simulink model "PID_ros"  (R2017b)
settings: Solver=FixedStepAuto  StartTime=0.0  StopTime=inf  FixedStep=dt_ros  RelTol=1e-3
values from neighbouring files (symbols this model uses):
  dt_ros = 0.02    [DOB_ros_adaptive_setup.m]    (also in DOB_ros_adaptive_w_kappa_setup.m; DOB_ros_setup.m)
  dt_ros_single = single(0.02)    [DOB_ros_adaptive_setup.m]    (also in DOB_ros_adaptive_w_kappa_setup.m; DOB_ros_setup.m)
  kc11 = single(0.3)    [DOB_ros_adaptive_setup.m]    (also in DOB_ros_adaptive_w_kappa_setup.m = single(1); DOB_ros_setup.m = kc1)
  kc12 = single(1)    [DOB_ros_adaptive_setup.m]    (also in DOB_ros_adaptive_w_kappa_setup.m = single(0); DOB_ros_setup.m = 1)
  kc2 = single(0.25)    [DOB_ros_adaptive_setup.m]    (also in DOB_ros_adaptive_w_kappa_setup.m = single(0.5); DOB_ros_setup.m = single(0.1))
  steering_ratio = 14.8    [DOB_ros_adaptive_setup.m]    (also in DOB_ros_adaptive_w_kappa_setup.m; DOB_ros_setup.m)
undefined symbols (not defined in the file or in its folder): Enable, SteeringWheelAngleCmd, SteeringWheelAngleVelocity
libraries: robotlib x4
settings Model: Creator=chen_tang  LastModifiedBy=root
settings OptimizationCC: PassReuseOutputArgsThreshold=0  MaxStackSize=64
settings DebuggingCC: ParameterTunabilityLossMsg=error
settings HardwareCC: ProdBitPerPointer=32  ProdBitPerSizeT=32  ProdBitPerPtrDiffT=32  ProdLargestAtomicFloat=None  ProdIntDivRoundTo=Undefined  ProdEndianess=Unspecified  ProdWordSize=32  ProdHWDeviceType=Generic->Unspecified (assume 32-bit Generic)  UseEmbeddedCoderFeatures=off
settings SFSimCC: MATLABDynamicMemAlloc=off
settings RTWCC: SystemTargetFile=ert.tlc  HardwareBoard=Robot Operating System (ROS)  TemplateMakefile=ert_default_tmf  GenerateReport=on  Toolchain=Catkin  LaunchReport=on  TargetLang=C++
settings CodeAppCC: ForceParamTrailComments=on  OperatorAnnotations=on  StateflowObjectComments=on  MATLABSourceComments=on
settings ERTTargetCC: ERTCustomFileBanners=off  SupportContinuousTime=on  SupportNonInlinedSFcns=on  RemoveResetFunc=off  ModelStepFunctionPrototypeControlCompliant=off

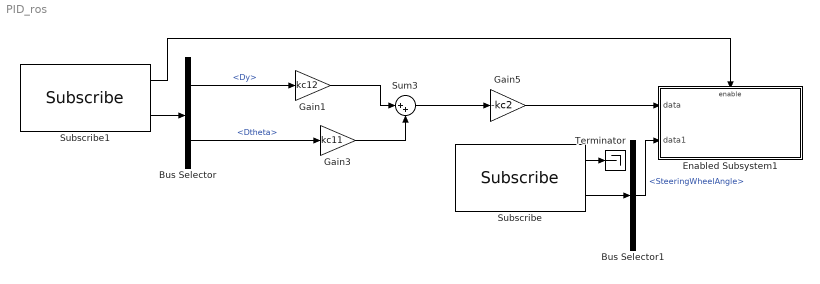
== system PID_ros ==
  Bus Selector : BusSelector  OutputSignals=Dy,Dtheta
  Bus Selector1 : BusSelector  OutputSignals=SteeringWheelAngle
  Enabled Subsystem1 : Subsystem  TreatAsAtomicUnit=on
  Gain1 : Gain  Gain=kc12  OutDataTypeStr=single
  Gain3 : Gain  Gain=kc11  OutDataTypeStr=single
  Gain5 : Gain  Gain=-kc2
  Subscribe : robotlib/Subscribe  SourceLibraryInfo=This block requires Robotics System Toolbox  topicSource=Specify your own  topic=/vehicle/steering_report  messageType=dbw_mkz_msgs/SteeringReport  sampleTime=-1  messageQueueLength=1
      settings: SourceProductBaseCode=RO
  Subscribe1 : robotlib/Subscribe  SourceLibraryInfo=This block requires Robotics System Toolbox  topicSource=Specify your own  topic=/tracking_info  messageType=controller/TrackingInfo  sampleTime=-1  messageQueueLength=1
      settings: SourceProductBaseCode=RO
  Sum3 : Sum  Inputs=|++  AccumDataTypeStr=single  OutDataTypeStr=single
  Terminator : Terminator
  wires:
  Subscribe1/2 -> Bus Selector/1
  Gain3/1 -> Sum3/2
  Subscribe1/1 -> Enabled Subsystem1/Enable
  Bus Selector/1 -> Gain1/1  "<Dy>"
  Bus Selector/2 -> Gain3/1  "<Dtheta>"
  Gain5/1 -> Enabled Subsystem1/1(data)
  Sum3/1 -> Gain5/1
  Subscribe/1 -> Terminator/1
  Subscribe/2 -> Bus Selector1/1
  Bus Selector1/1 -> Enabled Subsystem1/2(data1)  "<SteeringWheelAngle>"
  Gain1/1 -> Sum3/1

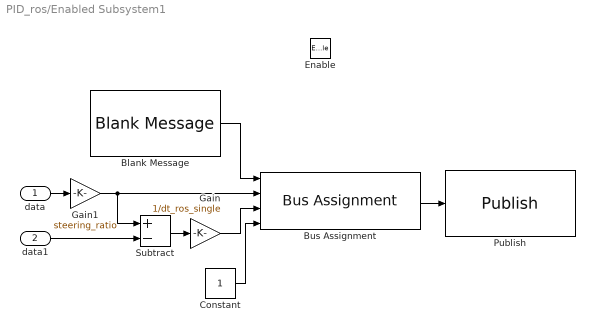
== system PID_ros/Enabled Subsystem1 ==
  data : Inport  OutDataTypeStr=single
  data1 : Inport  Port=2  OutDataTypeStr=single
  Enable : EnablePort
  Blank Message : robotlib/Blank Message  SourceLibraryInfo=This block requires Robotics System Toolbox  messageType=dbw_mkz_msgs/SteeringCmd  SampleTime=dt_ros
      settings: SourceProductBaseCode=RO
  Bus Assignment : BusAssignment  AssignedSignals=SteeringWheelAngleCmd,SteeringWheelAngleVelocity,Enable
  Constant : Constant  OutDataTypeStr=boolean
  Gain : Gain  Gain=1/dt_ros_single  ParamDataTypeStr=single  OutDataTypeStr=single
  Gain1 : Gain  Gain=steering_ratio  ParamDataTypeStr=single  OutDataTypeStr=single
  Publish : robotlib/Publish  SourceLibraryInfo=This block requires Robotics System Toolbox  topicSource=Specify your own  topic=/vehicle/steering_cmd  messageType=dbw_mkz_msgs/SteeringCmd  messageQueueLength=1
      settings: SourceProductBaseCode=RO
  Subtract : Sum  Inputs=+-  AccumDataTypeStr=single  OutDataTypeStr=single
  wires:
  Bus Assignment/1 -> Publish/1
  data/1 -> Gain1/1
  Blank Message/1 -> Bus Assignment/1
  data1/1 -> Subtract/2
  Subtract/1 -> Gain/1
  Gain/1 -> Bus Assignment/3
  Gain1/1 -> Subtract/1, Bus Assignment/2
  Constant/1 -> Bus Assignment/4
